simulink model "TrafficLight"  (R2021a)
settings: Solver=VariableStepAuto  StartTime=0.0  StopTime=20  RelTol=1e-3
settings Model: Creator=pc  LastModifiedBy=pc

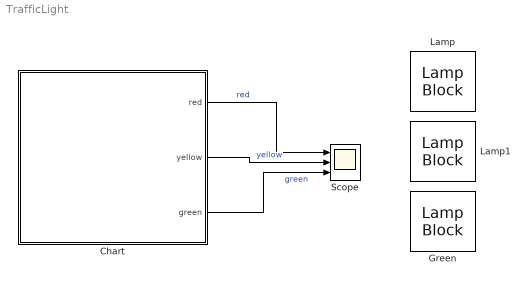
== system TrafficLight ==
  Chart : Stateflow chart  TreatAsAtomicUnit=on
  Green : LampBlock
  Lamp : LampBlock
  Lamp1 : LampBlock
  Scope : Scope  NumInputPorts=3
  wires:
  Chart/1(red) -> Scope/1  "red"
  Chart/3(green) -> Scope/3  "green"
  Chart/2(yellow) -> Scope/2  "yellow"

== stateflow chart TrafficLight/Chart ==
  state Stop
    entry:
    red = 1;
    yellow = 0;
    green = 0;
  state PrepareToStop
    entry:
    red = 0;
    yellow = 1;
    green = 0;
  state Go
    entry:
    red = 0;
    yellow = 0;
    green = 1;
  (default) -> Stop
  Stop -> (junction 26)
  (junction 26) -> (junction 29) : after(3,sec)
  PrepareToStop -> Stop : after(3,sec)
  Go -> PrepareToStop : after(5,sec)
  (junction 29) -> Go
  data: red output =1; yellow output; green output =0
